simulink model "validation_gate_debugging"  (Simulink 7.6)
settings: Solver=FixedStepDiscrete  StartTime=0.0  StopTime=0  RelTol=1e-3
libraries: vipanalysis x1
settings Model: Creator=Thing 1  LastModifiedBy=auvt
settings OptimizationCC: OptimizeModelRefInitCode=on
settings RTWCC: SystemTargetFile=ert.tlc  GenCodeOnly=on  TemplateMakefile=ert_default_tmf  Description=Real-Time Workshop Embedded Coder  GenerateReport=on  ProcessScript=ert_make_rtw_hook  IncludeHyperlinkInReport=on  LaunchReport=on  TargetLang=C++
settings CodeAppCC: IgnoreCustomStorageClasses=off
settings ERTTargetCC: MultiwordLength=2048  GenerateSampleERTMain=on  IncludeMdlTerminateFcn=off  ERTCustomFileTemplate=example_file_process.tlc  ConvertIfToSwitch=off

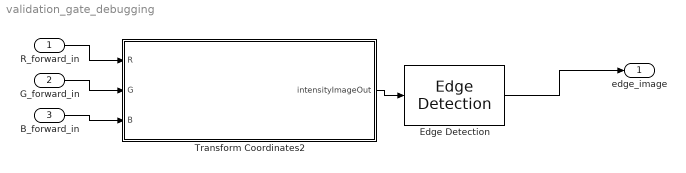
== system validation_gate_debugging ==
  R_forward_in : Inport  PortDimensions=Forward_Camera_Dimensions
  G_forward_in : Inport  Port=2  PortDimensions=Forward_Camera_Dimensions
  B_forward_in : Inport  Port=3  PortDimensions=Forward_Camera_Dimensions
  Edge Detection : vipanalysis/Edge Detection  DialogController=vipDDGCreate  DialogControllerArgs=DataTag0  method=Sobel  outputType=Binary image  userDefinedThreshold=off  thresholdSource=Specify via dialog  threshold=20  thresholdTuning=3  edgeThinning=on  threshold_canny=[0.25 0.60]  autoPercent=70  sigma=1  roundingMode=Floor  overflowMode=off
  Transform Coordinates2 : Stateflow chart  TreatAsAtomicUnit=on  SystemSampleTime=[1/30 0]
  edge_image : Outport
  wires:
  Transform Coordinates2/1(intensityImageOut) -> Edge Detection/1
  R_forward_in/1 -> Transform Coordinates2/1(R)
  G_forward_in/1 -> Transform Coordinates2/2(G)
  B_forward_in/1 -> Transform Coordinates2/3(B)
  Edge Detection/1 -> edge_image/1

== matlab function Transform Coordinates2 ==
  data: R input double; G input double; intensityImageOut output double; B input double
function intensityImageOut  = makeIntensity(R, G, B)

intensityImageOut = R + G + B;
intensityImageOut = intensityImageOut/max(max(max(intensityImageOut)));

%{

[rows, cols] = size(R);

for r = 1:rows
    for c = 1:cols
        
        if( intensityImageOut(r,c) == 0 )
            intensityImageOut(r,c) = 0;
        else
            intensityImageOut(r,c) = intensityImageOut(r,c)/max(max(intensityImageOut));
        end
    end
end

return




%}
